simulink model "ACC"  (R2025a)
settings: Solver=VariableStepAuto  StartTime=0.0  StopTime=80.0  RelTol=1e-3
model workspace (MAT data in the model file):
  Ts = 0.1
  default_spacing = 5
  max_ac = 2
  min_ac = -3
  time_gap = 2
  v0_lead = 25
  v0_self = 20
  v_set = 30
  verr_gain = 0.5
  vx_gain = 0.4
  x0_lead = 50
  x0_self = 0
  xerr_gain = 0.2
settings Model: Creator=howardchueh  LastModifiedBy=howardchueh

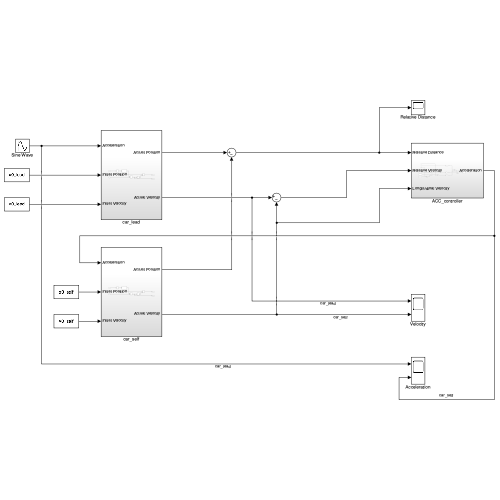
[thumbnail: Simulink's stored preview of the top-level diagram]
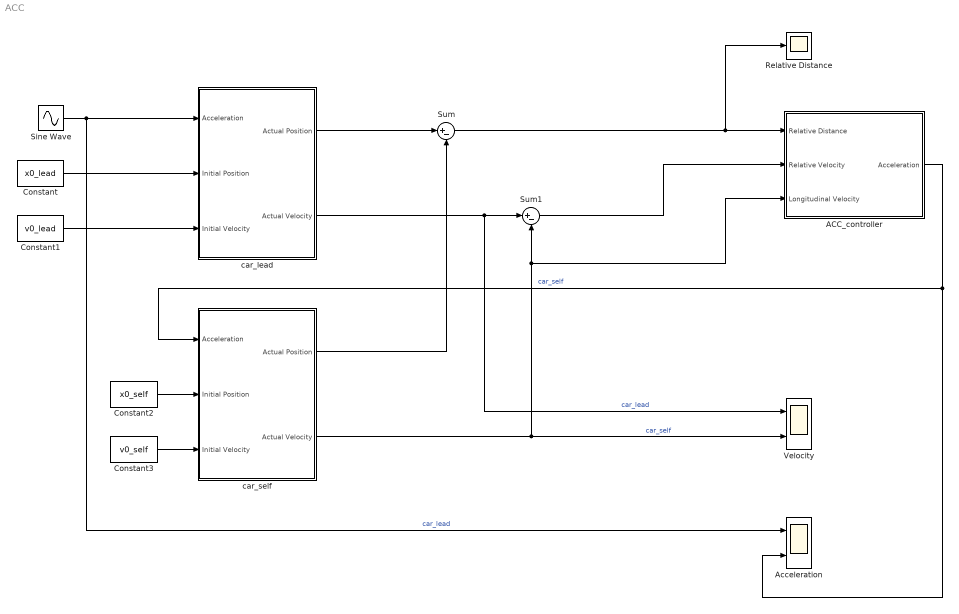
== system ACC ==
  ACC_controller : Subsystem
  Acceleration : Scope  NumInputPorts=2
      settings: ActiveDisplayYMinimum=-1.1819695345985441  ActiveDisplayYMaximum=2.3535521705109494  YLabel=m/s^2
  Constant : Constant  Value=x0_lead
  Constant1 : Constant  Value=v0_lead
  Constant2 : Constant  Value=x0_self
  Constant3 : Constant  Value=v0_self
  Relative Distance : Scope
      settings: ActiveDisplayYMinimum=47.44206933006987  ActiveDisplayYMaximum=73.021376029371169  YLabel=m  DataLoggingVariableName=ScopeData2
  Sine Wave : Sin  Amplitude=0.6  Frequency=0.2  SampleTime=0
  Sum : Sum  Inputs=|+-
  Sum1 : Sum  Inputs=|+-
  Velocity : Scope  NumInputPorts=2
      settings: ActiveDisplayYMinimum=18.6294073648771  ActiveDisplayYMaximum=32.335333716106121  YLabel=m/s
  car_lead : Subsystem
  car_self : Subsystem
  wires:
  Constant/1 -> car_lead/2(Initial Position)
  Sine Wave/1 -> Acceleration/1, car_lead/1(Acceleration)  "car_lead"
  Constant1/1 -> car_lead/3(Initial Velocity)
  car_lead/1(Actual Position) -> Sum/1
  Sum/1 -> Relative Distance/1, ACC_controller/1(Relative Distance)
  car_lead/2(Actual Velocity) -> Velocity/1, Sum1/1  "car_lead"
  Sum1/1 -> ACC_controller/2(Relative Velocity)
  car_self/1(Actual Position) -> Sum/2
  car_self/2(Actual Velocity) -> Velocity/2, ACC_controller/3(Longitudinal Velocity), Sum1/2  "car_self"
  Constant2/1 -> car_self/2(Initial Position)
  Constant3/1 -> car_self/3(Initial Velocity)
  ACC_controller/1(Acceleration) -> car_self/1(Acceleration), Acceleration/2  "car_self"

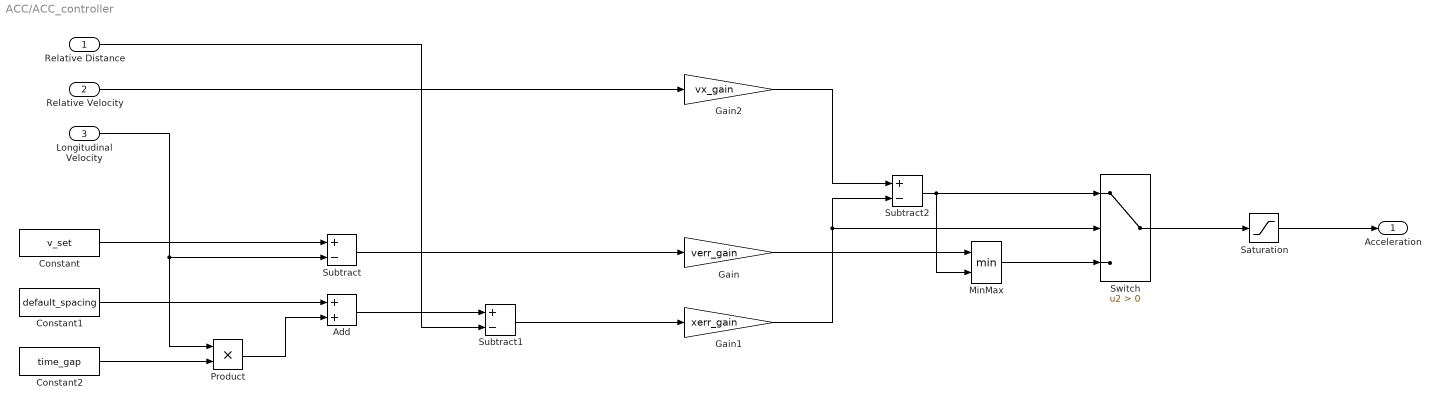
== system ACC/ACC_controller ==
  Relative Distance : Inport
  Relative Velocity : Inport  Port=2
  Longitudinal Velocity : Inport  Port=3
  Add : Sum
  Constant : Constant  Value=v_set
  Constant1 : Constant  Value=default_spacing
  Constant2 : Constant  Value=time_gap
  Gain : Gain  Gain=verr_gain
  Gain1 : Gain  Gain=xerr_gain
  Gain2 : Gain  Gain=vx_gain
  MinMax : MinMax  Inputs=2
  Product : Product
  Saturation : Saturate  UpperLimit=2  LowerLimit=-3
  Subtract : Sum  Inputs=+-
  Subtract1 : Sum  Inputs=+-
  Subtract2 : Sum  Inputs=+-
  Switch : Switch  Criteria=u2 > Threshold  SaturateOnIntegerOverflow=off  InputSameDT=off
  Acceleration : Outport
  wires:
  Constant2/1 -> Product/2
  Longitudinal Velocity/1 -> Subtract/2, Product/1
  Constant1/1 -> Add/1
  Product/1 -> Add/2
  Constant/1 -> Subtract/1
  Add/1 -> Subtract1/1
  Relative Distance/1 -> Subtract1/2
  Subtract/1 -> Gain/1
  Subtract1/1 -> Gain1/1
  Relative Velocity/1 -> Gain2/1
  Gain2/1 -> Subtract2/1
  Gain1/1 -> Subtract2/2, Switch/2
  Subtract2/1 -> MinMax/2, Switch/1
  MinMax/1 -> Switch/3
  Gain/1 -> MinMax/1
  Switch/1 -> Saturation/1
  Saturation/1 -> Acceleration/1

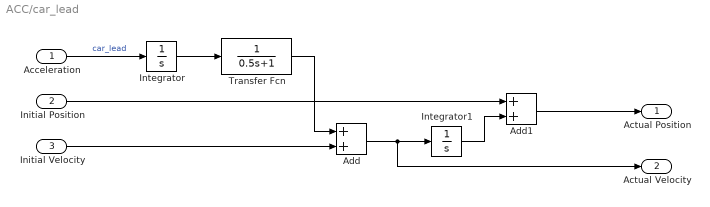
== system ACC/car_lead ==
  Acceleration : Inport
  Initial Position : Inport  Port=2
  Initial Velocity : Inport  Port=3
  Add : Sum
  Add1 : Sum
  Integrator : Integrator
  Integrator1 : Integrator
  Transfer Fcn : TransferFcn  Denominator=[0.5 1]
  Actual Position : Outport
  Actual Velocity : Outport  Port=2
  wires:
  Acceleration/1 -> Integrator/1  "car_lead"
  Integrator/1 -> Transfer Fcn/1
  Add/1 -> Actual Velocity/1, Integrator1/1
  Initial Velocity/1 -> Add/2
  Transfer Fcn/1 -> Add/1
  Initial Position/1 -> Add1/1
  Integrator1/1 -> Add1/2
  Add1/1 -> Actual Position/1

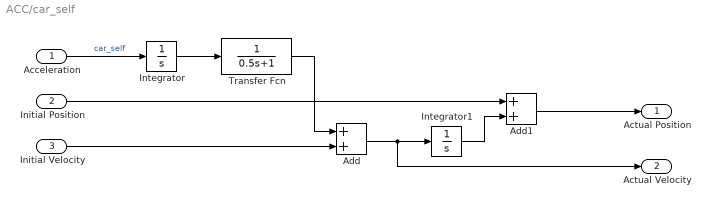
== system ACC/car_self ==
  Acceleration : Inport
  Initial Position : Inport  Port=2
  Initial Velocity : Inport  Port=3
  Add : Sum
  Add1 : Sum
  Integrator : Integrator
  Integrator1 : Integrator
  Transfer Fcn : TransferFcn  Denominator=[0.5 1]
  Actual Position : Outport
  Actual Velocity : Outport  Port=2
  wires:
  Acceleration/1 -> Integrator/1  "car_self"
  Integrator/1 -> Transfer Fcn/1
  Add/1 -> Actual Velocity/1, Integrator1/1
  Initial Velocity/1 -> Add/2
  Transfer Fcn/1 -> Add/1
  Initial Position/1 -> Add1/1
  Integrator1/1 -> Add1/2
  Add1/1 -> Actual Position/1
